simulink model "Hsp"  (Simulink 4.00)
settings: Solver=ode23t  StartTime=0  StopTime=70  FixedStep=0.01  RelTol=1e-3
PreLoadFcn:
  |  Control;HspInit;
values from neighbouring files (symbols this model uses):
  Cep = 1.67    [HspInit.m]    (also in hsp_data.mat)
  Cev = 50.0    (= 50)    [HspInit.m]    (also in hsp_data.mat)
  Cla = 19.23    [HspInit.m]    (also in hsp_data.mat)
  Cpa = 0.76    [HspInit.m]    (also in hsp_data.mat)
  Cpp = 5.80    (= 5.8)    [HspInit.m]    (also in hsp_data.mat)
  Cpv = 25.37    [HspInit.m]    (also in hsp_data.mat)
  Cra = 31.25    [HspInit.m]    (also in hsp_data.mat)
  Csa = 0.28    [HspInit.m]    (also in hsp_data.mat = 0.88)
  Csp = 2.05    [HspInit.m]    (also in hsp_data.mat)
  Csv = 61.11    [HspInit.m]    (also in hsp_data.mat)
  Dx = [  2     2     2     2    5      5        2   0.2 ]'    [Control.m]    (also in hsp_control.mat = [2 2 2 2 5 5 2 0.2])
  fcs0 = 25    [Control.m]    (also in hsp_control.mat)
  fes0 = 16.11    [Control.m]    (also in hsp_control.mat)
  fes1 = 2.10    (= 2.1)    [Control.m]    (also in hsp_control.mat)
  fesmin = 2.66    [Control.m]    (also in hsp_control.mat)
  fev0 = 3.2    [Control.m]    (also in hsp_control.mat)
  fev1 = 6.3    [Control.m]    (also in hsp_control.mat)
  fmax = 47.78    [Control.m]    (also in hsp_control.mat)
  fmin = 2.52    [Control.m]    (also in hsp_control.mat)
  Gx = [0.475 0.282  0.695 0.53 -265.4 -132.5  -0.13 0.09]'    [Control.m]    (also in hsp_control.mat = [0.475 0.282 0.695 0.53 -265.4 -132.5 -0.13 0.09])
  initx = [2.392 1.412  2.49  0.78 1435.4  1537    0.58   0]'    [Control.m]    (also in hsp_control.mat = [2.392 1.412 2.49 0.78 1400 1500 0.58 0])
  ka = 11.758    [Control.m]    (also in hsp_control.mat)
  KElv = 0.014    [HspInit.m]    (also in hsp_data.mat)
  KErv = 0.011    [HspInit.m]    (also in hsp_data.mat)
  kes = 0.0675    [Control.m]    (also in hsp_control.mat)
  kev = 7.06    [Control.m]    (also in hsp_control.mat)
  KRlv = 3.75e-4    (= 0.000375)    [HspInit.m]    (also in hsp_data.mat)
  KRrv = 1.4e-3    (= 0.0014)    [HspInit.m]    (also in hsp_data.mat)
  ksys = 0.075    [HspInit.m]    (also in hsp_data.mat)
  Lpa = 0.18e-3    (= 0.00018)    [HspInit.m]    (also in hsp_data.mat)
  Lsa = 0.22e-3    (= 0.00022)    [HspInit.m]    (also in hsp_data.mat)
  P0lv = 1.5    [HspInit.m]    (also in hsp_data.mat)
  P0rv = 1.5    [HspInit.m]    (also in hsp_data.mat)
  Pn = 92    [Control.m]    (also in hsp_control.mat)
  Rev = 0.016    [HspInit.m]    (also in hsp_data.mat)
  Rla = 25e-3    (= 0.025)    [HspInit.m]    (also in hsp_data.mat)
  Rpa = 0.023    [HspInit.m]    (also in hsp_data.mat)
  Rpp = 0.0894    [HspInit.m]    (also in hsp_data.mat)
  Rpv = 0.0056    [HspInit.m]    (also in hsp_data.mat)
  Rra = 2.5e-3    (= 0.0025)    [HspInit.m]    (also in hsp_data.mat)
  Rsa = 0.06    [HspInit.m]    (also in hsp_data.mat)
  Rsv = 0.038    [HspInit.m]    (also in hsp_data.mat)
  toup = 2.076    [Control.m]    (also in hsp_control.mat)
  toux = [  8     8     6     6    20     20       2   1.5 ]'    [Control.m]    (also in hsp_control.mat = [8 8 6 6 20 20 2 1.5])
  touz = 6.37    [Control.m]    (also in hsp_control.mat)
  Tsys0 = 0.5    [HspInit.m]    (also in hsp_data.mat)
  Vt = 5300    [HspInit.m]    (also in hsp_data.mat)
  Vuep = 336.6    [HspInit.m]    (also in hsp_data.mat)
  Vula = 25    [HspInit.m]    (also in hsp_data.mat)
  Vulv = 16.77    [HspInit.m]    (also in hsp_data.mat)
  Vupa = 0    [HspInit.m]    (also in hsp_data.mat)
  Vupp = 123    [HspInit.m]    (also in hsp_data.mat)
  Vupv = 120    [HspInit.m]    (also in hsp_data.mat)
  Vura = 25    [HspInit.m]    (also in hsp_data.mat)
  Vurv = 40.8    [HspInit.m]    (also in hsp_data.mat)
  Vusa = 0    [HspInit.m]    (also in hsp_data.mat)
  Vusp = 274.4    [HspInit.m]    (also in hsp_data.mat)
libraries: simulink3 x1
CloseFcn:
  | close(findobj(allchild(0),'flat','name','HSP Data Center'));close(findobj(allchild(0),'flat','name','HSP Control Center'))
settings Model: SaveOutput=off  InitialState=xFinal  SaveFinalState=on  LimitDataPoints=off  ExtModeTrigMode=oneshot  ExtModeArmWhenConnect=off  BlockReductionOpt=off

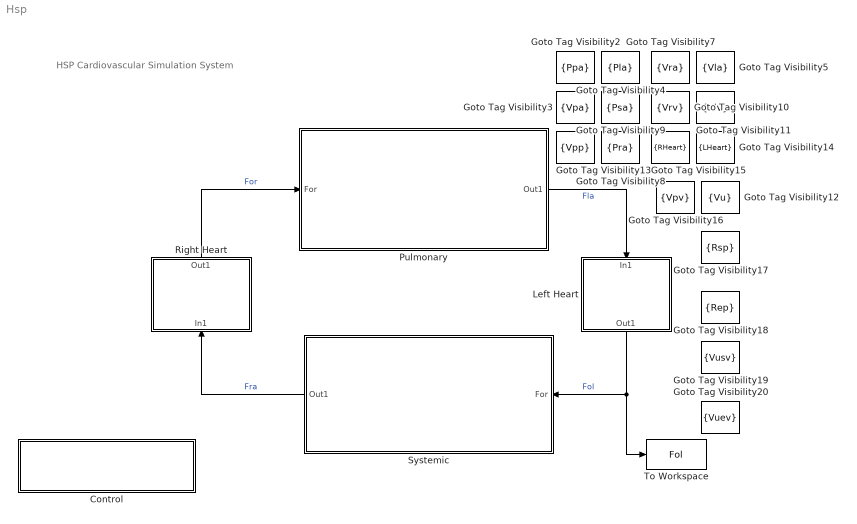
== system Hsp ==
  note: HSP
      | Cardiovascular Simulation System
  Control : Subsystem
      settings: RTWFcnNameOpts=Auto  RTWFileNameOpts=Auto
      mask Display: disp('ANALYSIS & CONTROL SYSTEM')
  Goto Tag Visibility10 : GotoTagVisibility  GotoTag=Vrv
  Goto Tag Visibility11 : GotoTagVisibility  GotoTag=Vlv
  Goto Tag Visibility12 : GotoTagVisibility  GotoTag=Vu
  Goto Tag Visibility13 : GotoTagVisibility  GotoTag=Vpp
  Goto Tag Visibility14 : GotoTagVisibility  GotoTag=LHeart
  Goto Tag Visibility15 : GotoTagVisibility  GotoTag=RHeart
  Goto Tag Visibility16 : GotoTagVisibility  GotoTag=Vpv
  Goto Tag Visibility17 : GotoTagVisibility  GotoTag=Rsp
  Goto Tag Visibility18 : GotoTagVisibility  GotoTag=Rep
  Goto Tag Visibility19 : GotoTagVisibility  GotoTag=Vusv
  Goto Tag Visibility2 : GotoTagVisibility  GotoTag=Ppa
  Goto Tag Visibility20 : GotoTagVisibility  GotoTag=Vuev
  Goto Tag Visibility3 : GotoTagVisibility  GotoTag=Vpa
  Goto Tag Visibility4 : GotoTagVisibility  GotoTag=Pla
  Goto Tag Visibility5 : GotoTagVisibility  GotoTag=Vla
  Goto Tag Visibility7 : GotoTagVisibility  GotoTag=Vra
  Goto Tag Visibility8 : GotoTagVisibility  GotoTag=Pra
  Goto Tag Visibility9 : GotoTagVisibility  GotoTag=Psa
  Left Heart : Subsystem  Orientation=down
      settings: RTWFcnNameOpts=Auto  RTWFileNameOpts=Auto
      mask Display: disp('LEFT HEART')
  Pulmonary : Subsystem
      settings: RTWFcnNameOpts=Auto  RTWFileNameOpts=Auto
      mask Display: disp('PULMONARY CIRCULATORY SYSTEM')
  Right Heart : Subsystem  Orientation=up
      settings: RTWFcnNameOpts=Auto  RTWFileNameOpts=Auto
      mask Display: disp('RIGHT HEART')
  Systemic : Subsystem  Orientation=left
      settings: RTWFcnNameOpts=Auto  RTWFileNameOpts=Auto
      mask Display: disp('SYSTEMIC CIRULATORY SYSTEM')
  To Workspace : ToWorkspace  VariableName=Fol  SampleTime=-1  SaveFormat=Array
  wires:
  Pulmonary/1(Out1) -> Left Heart/1(In1)  "Fla"
  Systemic/1(Out1) -> Right Heart/1(In1)  "Fra"
  Left Heart/1(Out1) -> Systemic/1(For), To Workspace/1  "Fol"
  Right Heart/1(Out1) -> Pulmonary/1(For)  "For"

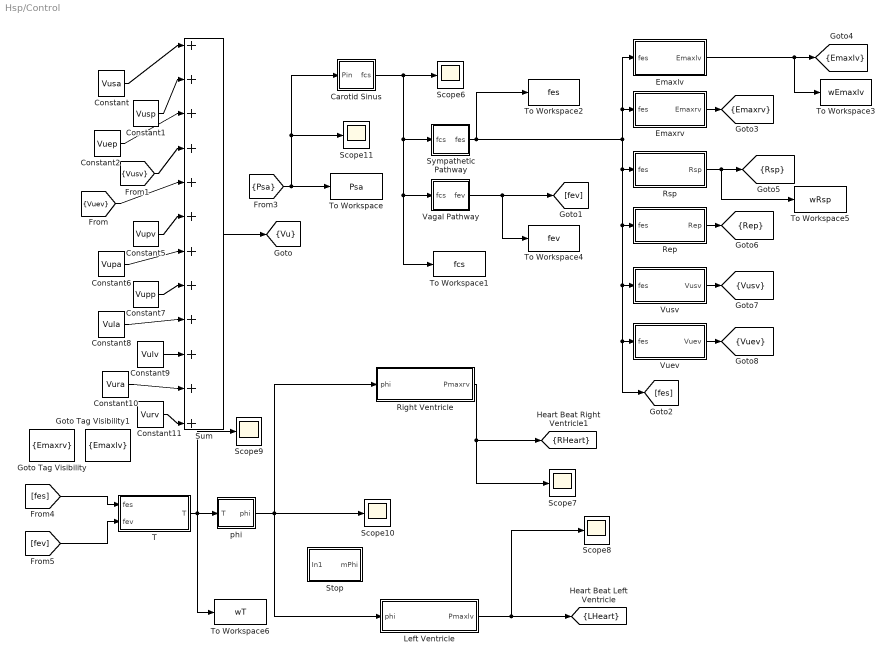
== system Hsp/Control ==
  Carotid Sinus : Subsystem
      settings: RTWFcnNameOpts=Auto  RTWFileNameOpts=Auto
  Constant : Constant  Value=Vusa
  Constant1 : Constant  Value=Vusp
  Constant10 : Constant  Value=Vura
  Constant11 : Constant  Value=Vurv
  Constant2 : Constant  Value=Vuep
  Constant5 : Constant  Value=Vupv
  Constant6 : Constant  Value=Vupa
  Constant7 : Constant  Value=Vupp
  Constant8 : Constant  Value=Vula
  Constant9 : Constant  Value=Vulv
  Emaxlv : Subsystem
      settings: RTWFcnNameOpts=Auto  RTWFileNameOpts=Auto
  Emaxrv : Subsystem
      settings: RTWFcnNameOpts=Auto  RTWFileNameOpts=Auto
  Goto Tag Visibility : GotoTagVisibility  GotoTag=Emaxrv
  Goto Tag Visibility1 : GotoTagVisibility  GotoTag=Emaxlv
  Left Ventricle : Subsystem
      settings: RTWFcnNameOpts=Auto  RTWFileNameOpts=Auto
  Rep : Subsystem
      settings: RTWFcnNameOpts=Auto  RTWFileNameOpts=Auto
  Right Ventricle : Subsystem
      settings: RTWFcnNameOpts=Auto  RTWFileNameOpts=Auto
  Rsp : Subsystem
      settings: RTWFcnNameOpts=Auto  RTWFileNameOpts=Auto
  Scope{6..11} (6 alike) : Scope
      Scope10 settings: TimeRange=auto  YMin=0  YMax=1  SaveToWorkspace=off  SaveName=ScopeData  LimitDataPoints=on  MaxDataPoints=5000
      Scope11 settings: TimeRange=auto  YMin=0  YMax=150  SaveToWorkspace=off  SaveName=ScopeData  LimitDataPoints=on  MaxDataPoints=5000
      Scope6 settings: TimeRange=auto  YMin=2.85  YMax=3.125  SaveToWorkspace=off  SaveName=ScopeData  LimitDataPoints=on  MaxDataPoints=5000
      Scope7 settings: TimeRange=auto  YMin=1.5  YMax=3.6  SaveToWorkspace=off  SaveName=ScopeData  LimitDataPoints=on  MaxDataPoints=5000
      Scope8 settings: TimeRange=auto  YMin=0  YMax=90  SaveToWorkspace=off  SaveName=ScopeData  LimitDataPoints=on  MaxDataPoints=5000
      Scope9 settings: TimeRange=auto  YMin=0.6  YMax=1.025  SaveToWorkspace=off  SaveName=ScopeData  LimitDataPoints=on  MaxDataPoints=5000
  Stop : Subsystem
      settings: RTWFcnNameOpts=Auto  RTWFileNameOpts=Auto
  Sum : Sum  Inputs=|++++++++++++  SaturateOnIntegerOverflow=on
  Sympathetic Pathway : Subsystem
      settings: RTWFcnNameOpts=Auto  RTWFileNameOpts=Auto
  T : Subsystem
      settings: RTWFcnNameOpts=Auto  RTWFileNameOpts=Auto
  To Workspace : ToWorkspace  VariableName=Psa  SampleTime=-1  SaveFormat=Array
  To Workspace1 : ToWorkspace  VariableName=fcs  SampleTime=-1  SaveFormat=Array
  To Workspace2 : ToWorkspace  VariableName=fes  SampleTime=-1  SaveFormat=Array
  To Workspace3 : ToWorkspace  VariableName=wEmaxlv  SampleTime=-1  SaveFormat=Array
  To Workspace4 : ToWorkspace  VariableName=fev  SampleTime=-1  SaveFormat=Array
  To Workspace5 : ToWorkspace  VariableName=wRsp  SampleTime=-1  SaveFormat=Array
  To Workspace6 : ToWorkspace  VariableName=wT  SampleTime=-1  SaveFormat=Array
  Vagal Pathway : Subsystem
      settings: RTWFcnNameOpts=Auto  RTWFileNameOpts=Auto
  Vuev : Subsystem
      settings: RTWFcnNameOpts=Auto  RTWFileNameOpts=Auto
  Vusv : Subsystem
      settings: RTWFcnNameOpts=Auto  RTWFileNameOpts=Auto
  phi : Subsystem
      settings: RTWFcnNameOpts=Auto  RTWFileNameOpts=Auto
  tag scope: Emaxlv=scoped, Emaxrv=scoped, LHeart=scoped, RHeart=scoped, Rep=scoped, Rsp=scoped, Vu=scoped, Vuev=scoped, Vusv=scoped
  wires:
  Sum/1 -> [Vu]
  Constant/1 -> Sum/1
  Constant2/1 -> Sum/3
  Constant1/1 -> Sum/2
  [Vusv] -> Sum/4
  [Vuev] -> Sum/5
  Constant5/1 -> Sum/6
  Constant6/1 -> Sum/7
  Constant7/1 -> Sum/8
  Constant8/1 -> Sum/9
  Constant9/1 -> Sum/10
  Constant10/1 -> Sum/11
  Constant11/1 -> Sum/12
  Carotid Sinus/1(fcs) -> Scope6/1, Sympathetic Pathway/1(fcs), Vagal Pathway/1(fcs), To Workspace1/1
  [fes] -> T/1(fes)
  [fev] -> T/2(fev)
  phi/1(phi) -> Scope10/1, Right Ventricle/1(phi), Left Ventricle/1(phi)
  Right Ventricle/1(Pmaxrv) -> [RHeart], Scope7/1
  Left Ventricle/1(Pmaxlv) -> [LHeart], Scope8/1
  Sympathetic Pathway/1(fes) -> Emaxlv/1(fes), Emaxrv/1(fes), Rsp/1(fes), Rep/1(fes), Vusv/1(fes), Vuev/1(fes), [fes], To Workspace2/1
  Emaxrv/1(Emaxrv) -> [Emaxrv]
  Rep/1(Rep) -> [Rep]
  Vusv/1(Vusv) -> [Vusv]
  Vuev/1(Vuev) -> [Vuev]
  Vagal Pathway/1(fev) -> [fev], To Workspace4/1
  Rsp/1(Rsp) -> [Rsp], To Workspace5/1
  [Psa] -> To Workspace/1, Scope11/1, Carotid Sinus/1(Pin)
  T/1(T) -> Scope9/1, To Workspace6/1, phi/1(T)
  Emaxlv/1(Emaxlv) -> [Emaxlv], To Workspace3/1

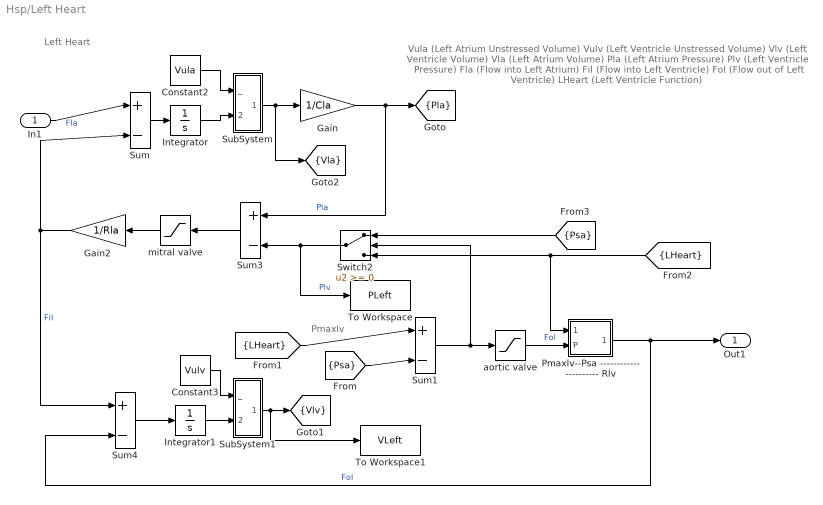
== system Hsp/Left Heart ==
  note: Left Heart
  note: Vula (Left Atrium Unstressed Volume)
      | Vulv (Left Ventricle Unstressed Volume)
      | Vlv (Left Ventricle Volume)
      | Vla (Left Atrium Volume)
      | Pla (Left Atrium Pressure)
      | Plv (Left Ventricle Pressure)
      | Fla (Flow into Left Atrium)
      | Fil (Flow into Left Ventricle)
      | Fol (Flow out of Left Ventricle)
      | LHeart (Left Ventricle Function)
  note: Pmaxlv
  In1 : Inport  Port=1
  Constant2 : Constant  Value=Vula
  Constant3 : Constant  Value=Vulv
  Gain : Gain  Gain=1/Cla  Multiplication=Element-wise(K.*u)  SaturateOnIntegerOverflow=on
  Gain2 : Gain  Orientation=left  Gain=1/Rla  Multiplication=Element-wise(K.*u)  SaturateOnIntegerOverflow=on
  Integrator : Integrator  ExternalReset=none  InitialConditionSource=internal  InitialCondition=0  LimitOutput=off  UpperSaturationLimit=inf  LowerSaturationLimit=-inf  ShowSaturationPort=off  ShowStatePort=off  AbsoluteTolerance=auto
  Integrator1 : Integrator  ExternalReset=none  InitialConditionSource=internal  InitialCondition=0  LimitOutput=off  UpperSaturationLimit=inf  LowerSaturationLimit=-inf  ShowSaturationPort=off  ShowStatePort=off  AbsoluteTolerance=auto
  Pmaxlv--Psa ---------------------- Rlv : Subsystem
      settings: RTWFcnNameOpts=Auto  RTWFileNameOpts=Auto
  SubSystem : Subsystem
      settings: RTWFcnNameOpts=Auto  RTWFileNameOpts=Auto
  SubSystem1 : Subsystem
      settings: RTWFcnNameOpts=Auto  RTWFileNameOpts=Auto
  Sum : Sum  Inputs=|+-  SaturateOnIntegerOverflow=on
  Sum1 : Sum  Inputs=|+-  SaturateOnIntegerOverflow=on
  Sum3 : Sum  Orientation=left  Inputs=+-  SaturateOnIntegerOverflow=on
  Sum4 : Sum  Inputs=+-  SaturateOnIntegerOverflow=on
  Switch2 : Switch  Orientation=left  Threshold=0
  To Workspace : ToWorkspace  VariableName=PLeft  SampleTime=-1  SaveFormat=Array
  To Workspace1 : ToWorkspace  VariableName=VLeft  SampleTime=-1  SaveFormat=Array
  aortic valve : Saturate  UpperLimit=inf  LowerLimit=0  LinearizeAsGain=on
  mitral valve : Saturate  Orientation=left  UpperLimit=inf  LowerLimit=0  LinearizeAsGain=on
  Out1 : Outport  Port=1
  tag scope: Pla=scoped, Vla=scoped, Vlv=scoped
  wires:
  In1/1 -> Sum/1  "Fla"
  Sum/1 -> Integrator/1
  [Psa] -> Sum1/2
  Gain/1 -> [Pla], Sum3/1  "Pla"
  Sum4/1 -> Integrator1/1
  Gain2/1 -> Sum/2, Sum4/1  "Fil"
  Pmaxlv--Psa ---------------------- Rlv/1(Flow) -> Out1/1, Sum4/2  "Fol"
  Constant2/1 -> SubSystem/1(_)
  Constant3/1 -> SubSystem1/1(_)
  SubSystem/1(Out) -> Gain/1, [Vla]
  [LHeart] -> Sum1/1
  Sum1/1 -> aortic valve/1, Switch2/2
  [Psa] -> Switch2/1
  mitral valve/1 -> Gain2/1
  [LHeart] -> Switch2/3, Pmaxlv--Psa ---------------------- Rlv/1(Pmax)
  aortic valve/1 -> Pmaxlv--Psa ---------------------- Rlv/2(P)  "Fol"
  Switch2/1 -> Sum3/2, To Workspace/1  "Plv"
  SubSystem1/1(Out) -> [Vlv], To Workspace1/1
  Integrator1/1 -> SubSystem1/2(+)
  Sum3/1 -> mitral valve/1
  Integrator/1 -> SubSystem/2(+)

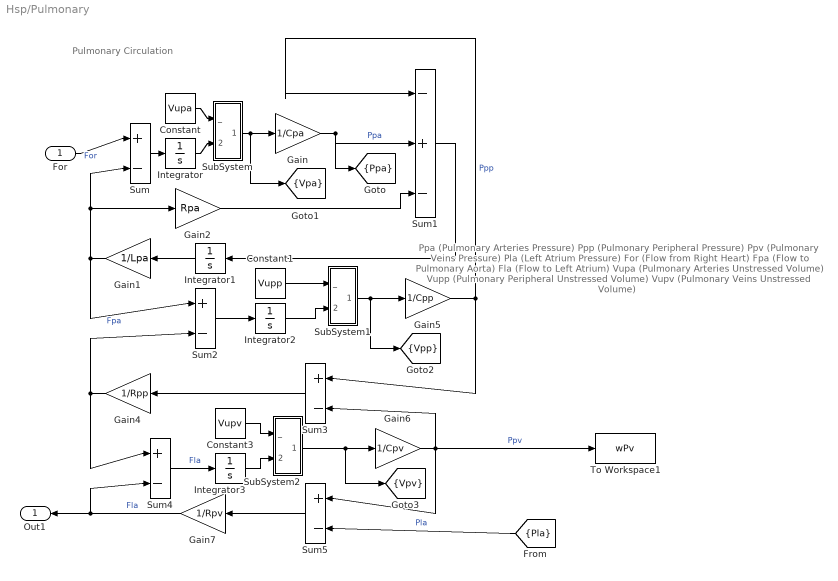
== system Hsp/Pulmonary ==
  note: Ppa (Pulmonary Arteries Pressure)
      | Ppp (Pulmonary Peripheral Pressure)
      | Ppv (Pulmonary Veins Pressure)
      | Pla (Left Atrium Pressure)
      | For (Flow from Right Heart)
      | Fpa (Flow to Pulmonary Aorta)
      | Fla (Flow to Left Atrium)
      | Vupa (Pulmonary Arteries Unstressed Volume)
      | Vupp (Pulmonary Peripheral Unstressed Volume)
      | Vupv (Pulmonary Veins Unstressed Volume)
  note: Pulmonary Circulation
  For : Inport  Port=1
  Constant : Constant  Value=Vupa
  Constant1 : Constant  Value=Vupp
  Constant3 : Constant  Value=Vupv
  Gain : Gain  Gain=1/Cpa  Multiplication=Element-wise(K.*u)  SaturateOnIntegerOverflow=on
  Gain1 : Gain  Orientation=left  Gain=1/Lpa  Multiplication=Element-wise(K.*u)  SaturateOnIntegerOverflow=on
  Gain2 : Gain  Gain=Rpa  Multiplication=Element-wise(K.*u)  SaturateOnIntegerOverflow=on
  Gain4 : Gain  Orientation=left  Gain=1/Rpp  Multiplication=Element-wise(K.*u)  SaturateOnIntegerOverflow=on
  Gain5 : Gain  Gain=1/Cpp  Multiplication=Element-wise(K.*u)  SaturateOnIntegerOverflow=on
  Gain6 : Gain  Gain=1/Cpv  Multiplication=Element-wise(K.*u)  SaturateOnIntegerOverflow=on
  Gain7 : Gain  Orientation=left  Gain=1/Rpv  Multiplication=Element-wise(K.*u)  SaturateOnIntegerOverflow=on
  Integrator : Integrator  ExternalReset=none  InitialConditionSource=internal  InitialCondition=100  LimitOutput=off  UpperSaturationLimit=inf  LowerSaturationLimit=-inf  ShowSaturationPort=off  ShowStatePort=off  AbsoluteTolerance=auto
  Integrator1 : Integrator  Orientation=left  ExternalReset=none  InitialConditionSource=internal  InitialCondition=0  LimitOutput=off  UpperSaturationLimit=inf  LowerSaturationLimit=-inf  ShowSaturationPort=off  ShowStatePort=off  AbsoluteTolerance=auto
  Integrator2 : Integrator  ExternalReset=none  InitialConditionSource=internal  InitialCondition=100  LimitOutput=off  UpperSaturationLimit=inf  LowerSaturationLimit=-inf  ShowSaturationPort=off  ShowStatePort=off  AbsoluteTolerance=auto
  Integrator3 : Integrator  ExternalReset=none  InitialConditionSource=internal  InitialCondition=0  LimitOutput=off  UpperSaturationLimit=inf  LowerSaturationLimit=-inf  ShowSaturationPort=off  ShowStatePort=off  AbsoluteTolerance=auto
  SubSystem : Subsystem
      settings: RTWFcnNameOpts=Auto  RTWFileNameOpts=Auto
  SubSystem1 : Subsystem
      settings: RTWFcnNameOpts=Auto  RTWFileNameOpts=Auto
  SubSystem2 : Subsystem
      settings: RTWFcnNameOpts=Auto  RTWFileNameOpts=Auto
  Sum : Sum  Inputs=|+-  SaturateOnIntegerOverflow=on
  Sum1 : Sum  Inputs=|-+-  SaturateOnIntegerOverflow=on
  Sum2 : Sum  Inputs=|+-  SaturateOnIntegerOverflow=on
  Sum3 : Sum  Orientation=left  Inputs=|+-  SaturateOnIntegerOverflow=on
  Sum4 : Sum  Inputs=|+-  SaturateOnIntegerOverflow=on
  Sum5 : Sum  Orientation=left  Inputs=|+-  SaturateOnIntegerOverflow=on
  To Workspace1 : ToWorkspace  VariableName=wPv  SampleTime=-1  SaveFormat=Array
  Out1 : Outport  Orientation=left  Port=1
  tag scope: Ppa=scoped, Vpa=scoped, Vpp=scoped, Vpv=scoped
  wires:
  For/1 -> Sum/1  "For"
  Sum/1 -> Integrator/1
  Integrator1/1 -> Gain1/1
  Sum1/1 -> Integrator1/1
  Gain2/1 -> Sum1/3
  Gain1/1 -> Sum/2, Gain2/1, Sum2/1  "Fpa"
  Sum2/1 -> Integrator2/1
  Gain5/1 -> Sum1/1, Sum3/1  "Ppp"
  Sum3/1 -> Gain4/1
  Gain4/1 -> Sum2/2, Sum4/1
  Sum5/1 -> Gain7/1
  Gain6/1 -> Sum3/2, Sum5/1, To Workspace1/1  "Ppv"
  [Pla] -> Sum5/2  "Pla"
  Sum4/1 -> Integrator3/1  "Fla"
  Gain/1 -> Sum1/2, [Ppa]  "Ppa"
  SubSystem/1(Out) -> Gain/1, [Vpa]
  SubSystem1/1(Out) -> Gain5/1, [Vpp]
  SubSystem2/1(Out) -> Gain6/1, [Vpv]
  Integrator/1 -> SubSystem/2(+)
  Constant/1 -> SubSystem/1(_)
  Constant1/1 -> SubSystem1/1(_)
  Integrator2/1 -> SubSystem1/2(+)
  Integrator3/1 -> SubSystem2/2(+)
  Gain7/1 -> Sum4/2, Out1/1  "Fla"
  Constant3/1 -> SubSystem2/1(_)

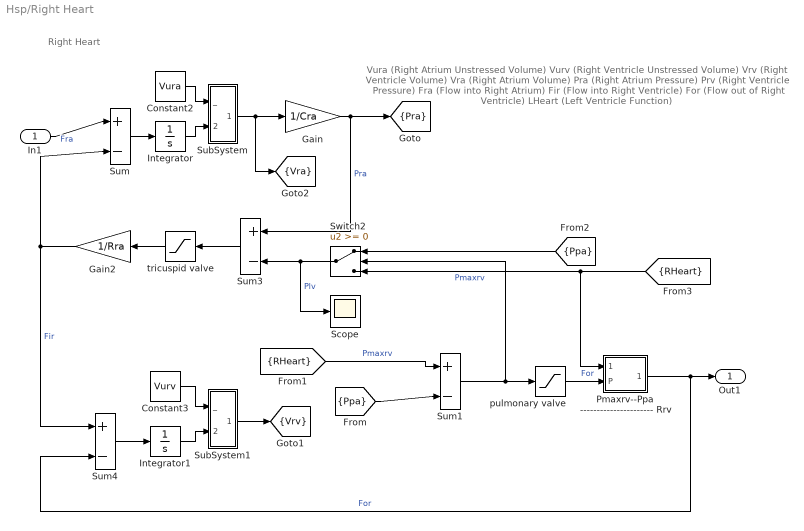
== system Hsp/Right Heart ==
  note: Right Heart
  note: Vura (Right Atrium Unstressed Volume)
      | Vurv (Right Ventricle Unstressed Volume)
      | Vrv (Right Ventricle Volume)
      | Vra (Right Atrium Volume)
      | Pra (Right Atrium Pressure)
      | Prv (Right Ventricle Pressure)
      | Fra (Flow into Right Atrium)
      | Fir (Flow into Right Ventricle)
      | For (Flow out of Right Ventricle)
      | LHeart (Left Ventricle Function)
  In1 : Inport  Port=1
  Constant2 : Constant  Value=Vura
  Constant3 : Constant  Value=Vurv
  Gain : Gain  Gain=1/Cra  Multiplication=Element-wise(K.*u)  SaturateOnIntegerOverflow=on
  Gain2 : Gain  Orientation=left  Gain=1/Rra  Multiplication=Element-wise(K.*u)  SaturateOnIntegerOverflow=on
  Integrator : Integrator  ExternalReset=none  InitialConditionSource=internal  InitialCondition=0  LimitOutput=off  UpperSaturationLimit=inf  LowerSaturationLimit=-inf  ShowSaturationPort=off  ShowStatePort=off  AbsoluteTolerance=auto
  Integrator1 : Integrator  ExternalReset=none  InitialConditionSource=internal  InitialCondition=0  LimitOutput=off  UpperSaturationLimit=inf  LowerSaturationLimit=-inf  ShowSaturationPort=off  ShowStatePort=off  AbsoluteTolerance=auto
  Pmaxrv--Ppa ---------------------- Rrv : Subsystem
      settings: RTWFcnNameOpts=Auto  RTWFileNameOpts=Auto
  Scope : Scope
      settings: TimeRange=auto  YMin=125  YMax=160  SaveToWorkspace=off  SaveName=ScopeData  LimitDataPoints=on  MaxDataPoints=5000
  SubSystem : Subsystem
      settings: RTWFcnNameOpts=Auto  RTWFileNameOpts=Auto
  SubSystem1 : Subsystem
      settings: RTWFcnNameOpts=Auto  RTWFileNameOpts=Auto
  Sum : Sum  Inputs=|+-  SaturateOnIntegerOverflow=on
  Sum1 : Sum  Inputs=|+-  SaturateOnIntegerOverflow=on
  Sum3 : Sum  Orientation=left  Inputs=+-  SaturateOnIntegerOverflow=on
  Sum4 : Sum  Inputs=+-  SaturateOnIntegerOverflow=on
  Switch2 : Switch  Orientation=left  Threshold=0
  pulmonary valve : Saturate  UpperLimit=inf  LowerLimit=0  LinearizeAsGain=on
  tricuspid valve : Saturate  Orientation=left  UpperLimit=inf  LowerLimit=0  LinearizeAsGain=on
  Out1 : Outport  Port=1
  tag scope: Pra=scoped, Vra=scoped, Vrv=scoped
  wires:
  In1/1 -> Sum/1  "Fra"
  Sum/1 -> Integrator/1
  [Ppa] -> Sum1/2
  Gain/1 -> [Pra], Sum3/1  "Pra"
  Gain2/1 -> Sum/2, Sum4/1  "Fir"
  Integrator/1 -> SubSystem/2(+)
  Constant2/1 -> SubSystem/1(_)
  SubSystem1/1(Out) -> [Vrv]
  SubSystem/1(Out) -> Gain/1, [Vra]
  Constant3/1 -> SubSystem1/1(_)
  Integrator1/1 -> SubSystem1/2(+)
  [RHeart] -> Sum1/1  "Pmaxrv"
  Sum1/1 -> pulmonary valve/1, Switch2/2
  [Ppa] -> Switch2/1
  tricuspid valve/1 -> Gain2/1
  pulmonary valve/1 -> Pmaxrv--Ppa ---------------------- Rrv/2(P)  "For"
  Pmaxrv--Ppa ---------------------- Rrv/1(Flow) -> Out1/1, Sum4/2  "For"
  [RHeart] -> Switch2/3, Pmaxrv--Ppa ---------------------- Rrv/1(Pmax)  "Pmaxrv"
  Sum4/1 -> Integrator1/1
  Sum3/1 -> tricuspid valve/1
  Switch2/1 -> Sum3/2, Scope/1  "Plv"

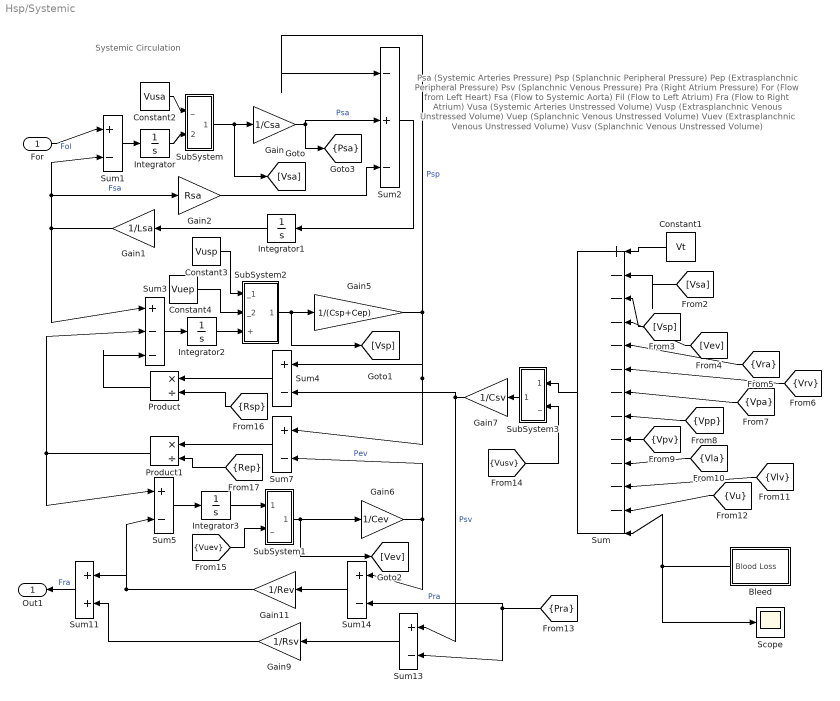
== system Hsp/Systemic ==
  note: Psa (Systemic Arteries Pressure)
      | Psp (Splanchnic Peripheral Pressure)
      | Pep (Extrasplanchnic Peripheral Pressure)
      | Psv (Splanchnic Venous Pressure)
      | Pra (Right Atrium Pressure)
      | For (Flow from Left Heart)
      | Fsa (Flow to Systemic Aorta)
      | Fil (Flow to Left Atrium)
      | Fra (Flow to Right Atrium)
      | Vusa (Systemic Arteries Unstressed Volume)
      | Vusp (Extrasplanchnic Venous Unstressed Volume)
      | Vuep (Splanchnic Venous Unstressed Volume)
      | Vuev (Extrasplanchnic Venous Unstressed Volume)
      | Vusv (Splanchnic Venous Unstressed Volume)
  note: Systemic Circulation
  For : Inport  Port=1
  Bleed : Subsystem  Orientation=left  mask{ulimit=0, rate=0, tstart=0}
      mask prompts: ulimit "Bleed Up Limit (ml)"; rate "Bleed Rate (ml/s)"; tstart "Bleed Start Time (s)"
      settings: RTWFcnNameOpts=Auto  RTWFileNameOpts=Auto
  Constant1 : Constant  Orientation=left  Value=Vt
  Constant2 : Constant  Value=Vusa
  Constant3 : Constant  Value=Vusp
  Constant4 : Constant  Value=Vuep
  Gain : Gain  Gain=1/Csa  Multiplication=Element-wise(K.*u)  SaturateOnIntegerOverflow=on
  Gain1 : Gain  Orientation=left  Gain=1/Lsa  Multiplication=Element-wise(K.*u)  SaturateOnIntegerOverflow=on
  Gain11 : Gain  Orientation=left  Gain=1/Rev  Multiplication=Element-wise(K.*u)  SaturateOnIntegerOverflow=on
  Gain2 : Gain  Gain=Rsa  Multiplication=Element-wise(K.*u)  SaturateOnIntegerOverflow=on
  Gain5 : Gain  Gain=1/(Csp+Cep)  Multiplication=Element-wise(K.*u)  SaturateOnIntegerOverflow=on
  Gain6 : Gain  Gain=1/Cev  Multiplication=Element-wise(K.*u)  SaturateOnIntegerOverflow=on
  Gain7 : Gain  Orientation=left  Gain=1/Csv  Multiplication=Element-wise(K.*u)  SaturateOnIntegerOverflow=on
  Gain9 : Gain  Orientation=left  Gain=1/Rsv  Multiplication=Element-wise(K.*u)  SaturateOnIntegerOverflow=on
  Integrator : Integrator  ExternalReset=none  InitialConditionSource=internal  InitialCondition=0  LimitOutput=off  UpperSaturationLimit=inf  LowerSaturationLimit=-inf  ShowSaturationPort=off  ShowStatePort=off  AbsoluteTolerance=auto
  Integrator1 : Integrator  Orientation=left  ExternalReset=none  InitialConditionSource=internal  InitialCondition=0  LimitOutput=off  UpperSaturationLimit=inf  LowerSaturationLimit=-inf  ShowSaturationPort=off  ShowStatePort=off  AbsoluteTolerance=auto
  Integrator2 : Integrator  ExternalReset=none  InitialConditionSource=internal  InitialCondition=0  LimitOutput=off  UpperSaturationLimit=inf  LowerSaturationLimit=-inf  ShowSaturationPort=off  ShowStatePort=off  AbsoluteTolerance=auto
  Integrator3 : Integrator  ExternalReset=none  InitialConditionSource=internal  InitialCondition=0  LimitOutput=off  UpperSaturationLimit=inf  LowerSaturationLimit=-inf  ShowSaturationPort=off  ShowStatePort=off  AbsoluteTolerance=auto
  Product : Product  Orientation=left  Inputs=*/  Multiplication=Element-wise(.*)  SaturateOnIntegerOverflow=on
  Product1 : Product  Orientation=left  Inputs=*/  Multiplication=Element-wise(.*)  SaturateOnIntegerOverflow=on
  Scope : Scope
      settings: TimeRange=auto  YMin=0  YMax=200  SaveToWorkspace=off  SaveName=ScopeData  LimitDataPoints=on  MaxDataPoints=5000
  SubSystem : Subsystem
      settings: RTWFcnNameOpts=Auto  RTWFileNameOpts=Auto
  SubSystem1 : Subsystem
      settings: RTWFcnNameOpts=Auto  RTWFileNameOpts=Auto
  SubSystem2 : Subsystem
      settings: RTWFcnNameOpts=Auto  RTWFileNameOpts=Auto
  SubSystem3 : Subsystem  Orientation=left
      settings: RTWFcnNameOpts=Auto  RTWFileNameOpts=Auto
  Sum : Sum  Orientation=left  Inputs=|+------------  SaturateOnIntegerOverflow=on
  Sum1 : Sum  Inputs=|+-  SaturateOnIntegerOverflow=on
  Sum11 : Sum  Orientation=left  Inputs=|++  SaturateOnIntegerOverflow=on
  Sum{4,7,13..14} (4 alike) : Sum  Orientation=left  Inputs=|+-  SaturateOnIntegerOverflow=on
  Sum2 : Sum  Inputs=|-+-  SaturateOnIntegerOverflow=on
  Sum3 : Sum  Inputs=|+--  SaturateOnIntegerOverflow=on
  Sum5 : Sum  Inputs=|+-  SaturateOnIntegerOverflow=on
  Out1 : Outport  Orientation=left  Port=1
  tag scope: Psa=scoped
  wires:
  For/1 -> Sum1/1  "Fol"
  Sum1/1 -> Integrator/1
  Integrator1/1 -> Gain1/1
  Sum2/1 -> Integrator1/1
  Gain2/1 -> Sum2/3
  Gain1/1 -> Sum1/2, Gain2/1, Sum3/1  "Fsa"
  Sum3/1 -> Integrator2/1
  Gain5/1 -> Sum2/1, Sum4/1, Sum7/1  "Psp"
  Product/1 -> Sum3/3
  Product1/1 -> Sum3/2, Sum5/1
  Integrator3/1 -> SubSystem1/1(+)
  SubSystem1/1(Out) -> Gain6/1, [Vev]
  Constant1/1 -> Sum/1
  [Vsa] -> Sum/2
  [Vsp] -> Sum/3
  [Vev] -> Sum/4
  [Vra] -> Sum/5
  [Vrv] -> Sum/6
  [Vpa] -> Sum/7
  [Vpp] -> Sum/8
  [Vpv] -> Sum/9
  [Vla] -> Sum/10
  [Vlv] -> Sum/11
  [Vu] -> Sum/12
  Integrator/1 -> SubSystem/2(+)
  SubSystem/1(Out) -> Gain/1, [Vsa]
  Integrator2/1 -> SubSystem2/3(+)
  SubSystem2/1(Out) -> Gain5/1, [Vsp]
  SubSystem3/1(Out) -> Gain7/1
  Sum13/1 -> Gain9/1
  Sum11/1 -> Out1/1  "Fra"
  Gain7/1 -> Sum4/2, Sum13/1  "Psv"
  Gain9/1 -> Sum11/2
  Gain6/1 -> Sum7/2, Sum14/1  "Pev"
  Sum14/1 -> Gain11/1
  [Pra] -> Sum13/2, Sum14/2  "Pra"
  Sum5/1 -> Integrator3/1
  Gain11/1 -> Sum11/1, Sum5/2
  Gain/1 -> Sum2/2, [Psa]  "Psa"
  Constant2/1 -> SubSystem/1(_)
  [Vuev] -> SubSystem1/2(_)
  Constant3/1 -> SubSystem2/1(_1)
  Constant4/1 -> SubSystem2/2(_2)
  Sum/1 -> SubSystem3/1(+)
  [Vusv] -> SubSystem3/2(_)
  Sum4/1 -> Product/1
  [Rsp] -> Product/2
  [Rep] -> Product1/2
  Sum7/1 -> Product1/1
  Bleed/1(Blood Loss) -> Sum/13, Scope/1

== system Hsp/Control/Carotid Sinus ==
  Pin : Inport  Port=1
  Fcn : Fcn  Expr=(fmin+fmax*exp((u-Pn)/ka))/(1+exp((u-Pn)/ka))
  Transfer Fcn : TransferFcn  Numerator=[touz 1]  Denominator=[toup 1]  Realization=auto  AbsoluteTolerance=auto
  fcs : Outport  Port=1
  wires:
  Pin/1 -> Transfer Fcn/1
  Transfer Fcn/1 -> Fcn/1
  Fcn/1 -> fcs/1

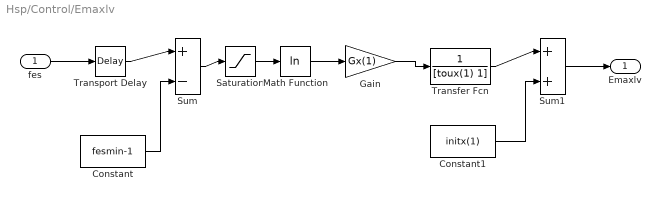
== system Hsp/Control/Emaxlv ==
  fes : Inport  Port=1
  Constant : Constant  Value=fesmin-1
  Constant1 : Constant  Value=initx(1)
  Gain : Gain  Gain=Gx(1)  Multiplication=Element-wise(K.*u)  SaturateOnIntegerOverflow=on
  Math Function : Math  Operator=log  OutputSignalType=auto
  Saturation : Saturate  UpperLimit=inf  LowerLimit=1  LinearizeAsGain=on
  Sum : Sum  Inputs=|+-  SaturateOnIntegerOverflow=on
  Sum1 : Sum  Inputs=|++  SaturateOnIntegerOverflow=on
  Transfer Fcn : TransferFcn  Numerator=[1]  Denominator=[toux(1) 1]  Realization=auto  AbsoluteTolerance=auto
  Transport Delay : TransportDelay  DelayTime=Dx(1)  InitialInput=0  BufferSize=1024  PadeOrder=0
  Emaxlv : Outport  Port=1
  wires:
  fes/1 -> Transport Delay/1
  Transport Delay/1 -> Sum/1
  Constant/1 -> Sum/2
  Sum/1 -> Saturation/1
  Saturation/1 -> Math Function/1
  Math Function/1 -> Gain/1
  Gain/1 -> Transfer Fcn/1
  Transfer Fcn/1 -> Sum1/1
  Sum1/1 -> Emaxlv/1
  Constant1/1 -> Sum1/2

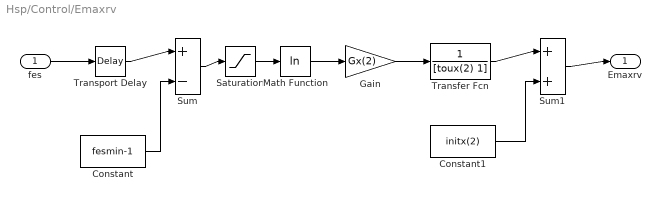
== system Hsp/Control/Emaxrv ==
  fes : Inport  Port=1
  Constant : Constant  Value=fesmin-1
  Constant1 : Constant  Value=initx(2)
  Gain : Gain  Gain=Gx(2)  Multiplication=Element-wise(K.*u)  SaturateOnIntegerOverflow=on
  Math Function : Math  Operator=log  OutputSignalType=auto
  Saturation : Saturate  UpperLimit=inf  LowerLimit=1  LinearizeAsGain=on
  Sum : Sum  Inputs=|+-  SaturateOnIntegerOverflow=on
  Sum1 : Sum  Inputs=|++  SaturateOnIntegerOverflow=on
  Transfer Fcn : TransferFcn  Numerator=[1]  Denominator=[toux(2) 1]  Realization=auto  AbsoluteTolerance=auto
  Transport Delay : TransportDelay  DelayTime=Dx(2)  InitialInput=0  BufferSize=1024  PadeOrder=0
  Emaxrv : Outport  Port=1
  wires:
  Constant1/1 -> Sum1/2
  Sum1/1 -> Emaxrv/1
  Transfer Fcn/1 -> Sum1/1
  Gain/1 -> Transfer Fcn/1
  Math Function/1 -> Gain/1
  Saturation/1 -> Math Function/1
  Sum/1 -> Saturation/1
  Constant/1 -> Sum/2
  Transport Delay/1 -> Sum/1
  fes/1 -> Transport Delay/1

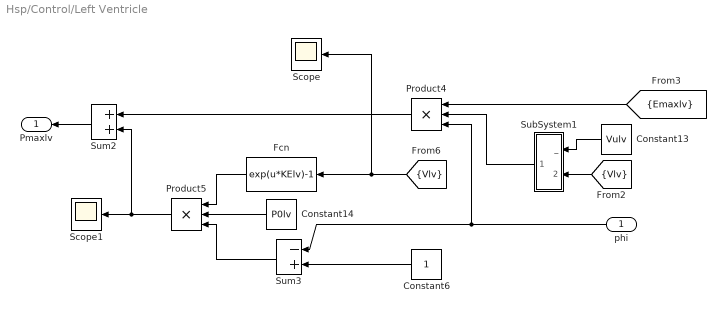
== system Hsp/Control/Left Ventricle ==
  phi : Inport  Orientation=left  Port=1
  Constant13 : Constant  Orientation=left  Value=Vulv
  Constant14 : Constant  Orientation=left  Value=P0lv
  Constant6 : Constant  Orientation=left  Value=1
  Fcn : Fcn  Orientation=left  Expr=exp(u*KElv)-1
  Product4 : Product  Orientation=left  Inputs=3  Multiplication=Element-wise(.*)  SaturateOnIntegerOverflow=on
  Product5 : Product  Orientation=left  Inputs=3  Multiplication=Element-wise(.*)  SaturateOnIntegerOverflow=on
  Scope : Scope
      settings: TimeRange=auto  YMin=0  YMax=250  SaveToWorkspace=off  SaveName=ScopeData  LimitDataPoints=on  MaxDataPoints=5000
  Scope1 : Scope
      settings: TimeRange=auto  YMin=0  YMax=35  SaveToWorkspace=off  LimitDataPoints=on  MaxDataPoints=5000
  SubSystem1 : Subsystem  Orientation=left
      settings: RTWFcnNameOpts=Auto  RTWFileNameOpts=Auto
  Sum2 : Sum  Orientation=left  Inputs=++  SaturateOnIntegerOverflow=on
  Sum3 : Sum  Orientation=left  Inputs=-+  SaturateOnIntegerOverflow=on
  Pmaxlv : Outport  Orientation=left  Port=1
  wires:
  Sum2/1 -> Pmaxlv/1
  Product4/1 -> Sum2/1
  Product5/1 -> Sum2/2, Scope1/1
  Fcn/1 -> Product5/1
  Constant14/1 -> Product5/2
  Sum3/1 -> Product5/3
  Constant6/1 -> Sum3/2
  Constant13/1 -> SubSystem1/1(_)
  [Vlv] -> SubSystem1/2(+)
  SubSystem1/1(Out) -> Product4/2
  phi/1 -> Sum3/1, Product4/3
  [Emaxlv] -> Product4/1
  [Vlv] -> Fcn/1, Scope/1

== system Hsp/Control/Rep ==
  fes : Inport  Port=1
  Constant : Constant  Value=fesmin-1
  Constant1 : Constant  Value=initx(4)
  Gain : Gain  Gain=Gx(4)  Multiplication=Element-wise(K.*u)  SaturateOnIntegerOverflow=on
  Math Function : Math  Operator=log  OutputSignalType=auto
  Saturation : Saturate  UpperLimit=inf  LowerLimit=1  LinearizeAsGain=on
  Sum : Sum  Inputs=|+-  SaturateOnIntegerOverflow=on
  Sum1 : Sum  Inputs=|++  SaturateOnIntegerOverflow=on
  Transfer Fcn : TransferFcn  Numerator=[1]  Denominator=[toux(4) 1]  Realization=auto  AbsoluteTolerance=auto
  Transport Delay : TransportDelay  DelayTime=Dx(4)  InitialInput=0  BufferSize=1024  PadeOrder=0
  Rep : Outport  Port=1
  wires:
  Constant1/1 -> Sum1/2
  Sum1/1 -> Rep/1
  Transfer Fcn/1 -> Sum1/1
  Gain/1 -> Transfer Fcn/1
  Math Function/1 -> Gain/1
  Saturation/1 -> Math Function/1
  Sum/1 -> Saturation/1
  Constant/1 -> Sum/2
  Transport Delay/1 -> Sum/1
  fes/1 -> Transport Delay/1

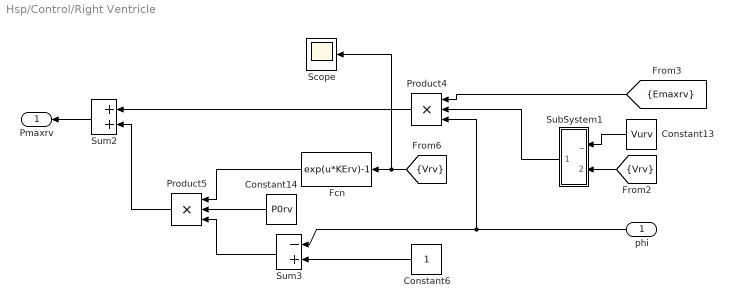
== system Hsp/Control/Right Ventricle ==
  phi : Inport  Orientation=left  Port=1
  Constant13 : Constant  Orientation=left  Value=Vurv
  Constant14 : Constant  Orientation=left  Value=P0rv
  Constant6 : Constant  Orientation=left  Value=1
  Fcn : Fcn  Orientation=left  Expr=exp(u*KErv)-1
  Product4 : Product  Orientation=left  Inputs=3  Multiplication=Element-wise(.*)  SaturateOnIntegerOverflow=on
  Product5 : Product  Orientation=left  Inputs=3  Multiplication=Element-wise(.*)  SaturateOnIntegerOverflow=on
  Scope : Scope
      settings: TimeRange=auto  YMin=45  YMax=85  SaveToWorkspace=off  SaveName=ScopeData  LimitDataPoints=on  MaxDataPoints=5000
  SubSystem1 : Subsystem  Orientation=left
      settings: RTWFcnNameOpts=Auto  RTWFileNameOpts=Auto
  Sum2 : Sum  Orientation=left  Inputs=++  SaturateOnIntegerOverflow=on
  Sum3 : Sum  Orientation=left  Inputs=-+  SaturateOnIntegerOverflow=on
  Pmaxrv : Outport  Orientation=left  Port=1
  wires:
  Constant6/1 -> Sum3/2
  Sum3/1 -> Product5/3
  Constant14/1 -> Product5/2
  Fcn/1 -> Product5/1
  Product5/1 -> Sum2/2
  Product4/1 -> Sum2/1
  Sum2/1 -> Pmaxrv/1
  [Emaxrv] -> Product4/1
  [Vrv] -> SubSystem1/2(+)
  Constant13/1 -> SubSystem1/1(_)
  SubSystem1/1(Out) -> Product4/2
  phi/1 -> Sum3/1, Product4/3
  [Vrv] -> Fcn/1, Scope/1

== system Hsp/Control/Rsp ==
  fes : Inport  Port=1
  Constant : Constant  Value=fesmin-1
  Constant1 : Constant  Value=initx(3)
  Gain : Gain  Gain=Gx(3)  Multiplication=Element-wise(K.*u)  SaturateOnIntegerOverflow=on
  Math Function : Math  Operator=log  OutputSignalType=auto
  Saturation : Saturate  UpperLimit=inf  LowerLimit=1  LinearizeAsGain=on
  Sum : Sum  Inputs=|+-  SaturateOnIntegerOverflow=on
  Sum1 : Sum  Inputs=|++  SaturateOnIntegerOverflow=on
  Transfer Fcn : TransferFcn  Numerator=[1]  Denominator=[toux(3) 1]  Realization=auto  AbsoluteTolerance=auto
  Transport Delay : TransportDelay  DelayTime=Dx(3)  InitialInput=0  BufferSize=1024  PadeOrder=0
  Rsp : Outport  Port=1
  wires:
  fes/1 -> Transport Delay/1
  Transport Delay/1 -> Sum/1
  Constant/1 -> Sum/2
  Sum/1 -> Saturation/1
  Saturation/1 -> Math Function/1
  Math Function/1 -> Gain/1
  Gain/1 -> Transfer Fcn/1
  Transfer Fcn/1 -> Sum1/1
  Sum1/1 -> Rsp/1
  Constant1/1 -> Sum1/2

== system Hsp/Control/Stop ==
  In1 : Inport  Port=1
  Clock : Clock
      settings: DisplayTime=off  Decimation=10
  Constant : Constant  Value=0
  Switch : Switch  Threshold=50
  mPhi : Outport  Port=1
  wires:
  In1/1 -> Switch/3
  Constant/1 -> Switch/1
  Switch/1 -> mPhi/1
  Clock/1 -> Switch/2

== system Hsp/Control/Sympathetic Pathway ==
  fcs : Inport  Port=1
  Constant : Constant  Value=fes1
  Gain : Gain  Gain=-kes  Multiplication=Element-wise(K.*u)  SaturateOnIntegerOverflow=on
  Gain1 : Gain  Gain=fes0-fes1  Multiplication=Element-wise(K.*u)  SaturateOnIntegerOverflow=on
  Math Function : Math  Operator=exp  OutputSignalType=auto
  Sum : Sum  Inputs=|++  SaturateOnIntegerOverflow=on
  fes : Outport  Port=1
  wires:
  Gain1/1 -> Sum/1
  Constant/1 -> Sum/2
  Sum/1 -> fes/1
  fcs/1 -> Gain/1
  Gain/1 -> Math Function/1
  Math Function/1 -> Gain1/1

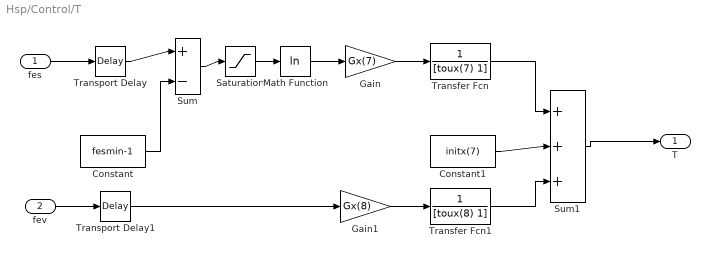
== system Hsp/Control/T ==
  fes : Inport  Port=1
  fev : Inport  Port=2
  Constant : Constant  Value=fesmin-1
  Constant1 : Constant  Value=initx(7)
  Gain : Gain  Gain=Gx(7)  Multiplication=Element-wise(K.*u)  SaturateOnIntegerOverflow=on
  Gain1 : Gain  Gain=Gx(8)  Multiplication=Element-wise(K.*u)  SaturateOnIntegerOverflow=on
  Math Function : Math  Operator=log  OutputSignalType=auto
  Saturation : Saturate  UpperLimit=inf  LowerLimit=1  LinearizeAsGain=on
  Sum : Sum  Inputs=|+-  SaturateOnIntegerOverflow=on
  Sum1 : Sum  Inputs=|+++  SaturateOnIntegerOverflow=on
  Transfer Fcn : TransferFcn  Numerator=[1]  Denominator=[toux(7) 1]  Realization=auto  AbsoluteTolerance=auto
  Transfer Fcn1 : TransferFcn  Numerator=[1]  Denominator=[toux(8) 1]  Realization=auto  AbsoluteTolerance=auto
  Transport Delay : TransportDelay  DelayTime=Dx(7)  InitialInput=0  BufferSize=1024  PadeOrder=0
  Transport Delay1 : TransportDelay  DelayTime=Dx(8)  InitialInput=0  BufferSize=1024  PadeOrder=0
  T : Outport  Port=1
  wires:
  fes/1 -> Transport Delay/1
  Transport Delay/1 -> Sum/1
  Constant/1 -> Sum/2
  Sum/1 -> Saturation/1
  Saturation/1 -> Math Function/1
  Math Function/1 -> Gain/1
  Gain/1 -> Transfer Fcn/1
  Transfer Fcn/1 -> Sum1/1
  Sum1/1 -> T/1
  Constant1/1 -> Sum1/2
  fev/1 -> Transport Delay1/1
  Transport Delay1/1 -> Gain1/1
  Gain1/1 -> Transfer Fcn1/1
  Transfer Fcn1/1 -> Sum1/3

== system Hsp/Control/Vagal Pathway ==
  fcs : Inport  Port=1
  Fcn : Fcn  Expr=(fev0+fev1*exp((u-fcs0)/kev))/(1+exp((u-fcs0)/kev))
  fev : Outport  Port=1
  wires:
  Fcn/1 -> fev/1
  fcs/1 -> Fcn/1

== system Hsp/Control/Vuev ==
  fes : Inport  Port=1
  Constant : Constant  Value=fesmin-1
  Constant1 : Constant  Value=initx(6)
  Gain : Gain  Gain=Gx(6)  Multiplication=Element-wise(K.*u)  SaturateOnIntegerOverflow=on
  Math Function : Math  Operator=log  OutputSignalType=auto
  Saturation : Saturate  UpperLimit=inf  LowerLimit=1  LinearizeAsGain=on
  Sum : Sum  Inputs=|+-  SaturateOnIntegerOverflow=on
  Sum1 : Sum  Inputs=|++  SaturateOnIntegerOverflow=on
  Transfer Fcn : TransferFcn  Numerator=[1]  Denominator=[toux(6) 1]  Realization=auto  AbsoluteTolerance=auto
  Transport Delay : TransportDelay  DelayTime=Dx(6)  InitialInput=0  BufferSize=1024  PadeOrder=0
  Vuev : Outport  Port=1
  wires:
  Constant1/1 -> Sum1/2
  Sum1/1 -> Vuev/1
  Transfer Fcn/1 -> Sum1/1
  Gain/1 -> Transfer Fcn/1
  Math Function/1 -> Gain/1
  Saturation/1 -> Math Function/1
  Sum/1 -> Saturation/1
  Constant/1 -> Sum/2
  Transport Delay/1 -> Sum/1
  fes/1 -> Transport Delay/1

== system Hsp/Control/Vusv ==
  fes : Inport  Port=1
  Constant : Constant  Value=fesmin-1
  Constant1 : Constant  Value=initx(5)
  Gain : Gain  Gain=Gx(5)  Multiplication=Element-wise(K.*u)  SaturateOnIntegerOverflow=on
  Math Function : Math  Operator=log  OutputSignalType=auto
  Saturation : Saturate  UpperLimit=inf  LowerLimit=1  LinearizeAsGain=on
  Sum : Sum  Inputs=|+-  SaturateOnIntegerOverflow=on
  Sum1 : Sum  Inputs=|++  SaturateOnIntegerOverflow=on
  Transfer Fcn : TransferFcn  Numerator=[1]  Denominator=[toux(5) 1]  Realization=auto  AbsoluteTolerance=auto
  Transport Delay : TransportDelay  DelayTime=Dx(5)  InitialInput=0  BufferSize=1024  PadeOrder=0
  Vusv : Outport  Port=1
  wires:
  fes/1 -> Transport Delay/1
  Transport Delay/1 -> Sum/1
  Constant/1 -> Sum/2
  Sum/1 -> Saturation/1
  Saturation/1 -> Math Function/1
  Math Function/1 -> Gain/1
  Gain/1 -> Transfer Fcn/1
  Transfer Fcn/1 -> Sum1/1
  Sum1/1 -> Vusv/1
  Constant1/1 -> Sum1/2

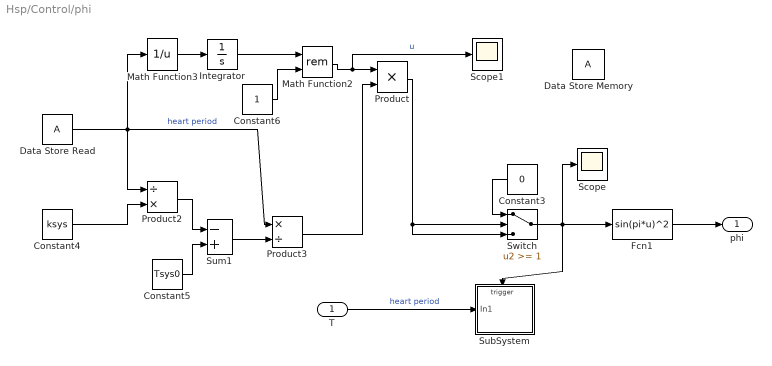
== system Hsp/Control/phi ==
  T : Inport  Port=1
  Constant3 : Constant  Orientation=left  Value=0
  Constant4 : Constant  Value=ksys
  Constant5 : Constant  Value=Tsys0
  Constant6 : Constant  Value=1
  Data Store Memory : DataStoreMemory  DataStoreName=A  InitialValue=initx(7)
  Data Store Read : DataStoreRead  DataStoreName=A  SampleTime=0
  Fcn1 : Fcn  Expr=sin(pi*u)^2
  Integrator : Integrator  ExternalReset=none  InitialConditionSource=internal  InitialCondition=0  LimitOutput=off  UpperSaturationLimit=inf  LowerSaturationLimit=-inf  ShowSaturationPort=off  ShowStatePort=off  AbsoluteTolerance=auto
  Math Function2 : Math  Operator=rem  OutputSignalType=auto
  Math Function3 : Math  Operator=reciprocal  OutputSignalType=auto
  Product : Product  Inputs=2  Multiplication=Element-wise(.*)  SaturateOnIntegerOverflow=on
  Product2 : Product  Inputs=/*  Multiplication=Element-wise(.*)  SaturateOnIntegerOverflow=on
  Product3 : Product  Inputs=*/  Multiplication=Element-wise(.*)  SaturateOnIntegerOverflow=on
  Scope : Scope
      settings: TimeRange=auto  YMin=0  YMax=1  SaveToWorkspace=off  SaveName=ScopeData  LimitDataPoints=on  MaxDataPoints=5000
  Scope1 : Scope
      settings: TimeRange=auto  YMin=5.55112e-017  YMax=1  SaveToWorkspace=off  SaveName=ScopeData  LimitDataPoints=on  MaxDataPoints=5000
  SubSystem : Subsystem  TreatAsAtomicUnit=on
      settings: RTWFcnNameOpts=Auto  RTWFileNameOpts=Auto
  Sum1 : Sum  Inputs=-+  SaturateOnIntegerOverflow=on
  Switch : Switch  Threshold=1
  phi : Outport  Port=1
  wires:
  Product3/1 -> Product/2
  Sum1/1 -> Product3/2
  Constant5/1 -> Sum1/2
  Product2/1 -> Sum1/1
  Constant4/1 -> Product2/2
  Constant3/1 -> Switch/1
  Product/1 -> Switch/2, Switch/3
  Fcn1/1 -> phi/1
  T/1 -> SubSystem/1(In1)  "heart period"
  Switch/1 -> Fcn1/1, SubSystem/Trigger, Scope/1
  Data Store Read/1 -> Product3/1, Product2/1, Math Function3/1  "heart period"
  Constant6/1 -> Math Function2/2
  Math Function2/1 -> Product/1, Scope1/1  "u"
  Math Function3/1 -> Integrator/1
  Integrator/1 -> Math Function2/1

== system Hsp/Left Heart/Pmaxlv--Psa ---------------------- Rlv ==
  Pmax : Inport  Port=1
  P : Inport  Port=2
  Gain : Gain  Gain=KRlv  Multiplication=Element-wise(K.*u)  SaturateOnIntegerOverflow=on
  Product : Product  Inputs=/*  Multiplication=Element-wise(.*)  SaturateOnIntegerOverflow=on
  Saturation : Saturate  UpperLimit=inf  LowerLimit=0.01  LinearizeAsGain=on
  Flow : Outport  Port=1
  wires:
  Pmax/1 -> Gain/1
  Gain/1 -> Saturation/1
  P/1 -> Product/2
  Saturation/1 -> Product/1
  Product/1 -> Flow/1

== system Hsp/Left Heart/SubSystem ==
  _ : Inport  Port=1
  + : Inport  Port=2
  Saturation : Saturate  UpperLimit=10000  LowerLimit=0  LinearizeAsGain=on
  Sum : Sum  Inputs=|-+  SaturateOnIntegerOverflow=on
  Out : Outport  Port=1
  wires:
  _/1 -> Sum/1
  +/1 -> Sum/2
  Sum/1 -> Saturation/1
  Saturation/1 -> Out/1

== system Hsp/Left Heart/SubSystem1 ==
  _ : Inport  Port=1
  + : Inport  Port=2
  Saturation : Saturate  UpperLimit=10000  LowerLimit=0  LinearizeAsGain=on
  Sum : Sum  Inputs=|-+  SaturateOnIntegerOverflow=on
  Out : Outport  Port=1
  wires:
  Saturation/1 -> Out/1
  Sum/1 -> Saturation/1
  +/1 -> Sum/2
  _/1 -> Sum/1

== system Hsp/Pulmonary/SubSystem ==
  _ : Inport  Port=1
  + : Inport  Port=2
  Saturation : Saturate  UpperLimit=10000  LowerLimit=0  LinearizeAsGain=on
  Sum : Sum  Inputs=|-+  SaturateOnIntegerOverflow=on
  Out : Outport  Port=1
  wires:
  _/1 -> Sum/1
  +/1 -> Sum/2
  Sum/1 -> Saturation/1
  Saturation/1 -> Out/1

== system Hsp/Pulmonary/SubSystem1 ==
  _ : Inport  Port=1
  + : Inport  Port=2
  Saturation : Saturate  UpperLimit=10000  LowerLimit=0  LinearizeAsGain=on
  Sum : Sum  Inputs=|-+  SaturateOnIntegerOverflow=on
  Out : Outport  Port=1
  wires:
  _/1 -> Sum/1
  +/1 -> Sum/2
  Sum/1 -> Saturation/1
  Saturation/1 -> Out/1

== system Hsp/Pulmonary/SubSystem2 ==
  _ : Inport  Port=1
  + : Inport  Port=2
  Saturation : Saturate  UpperLimit=10000  LowerLimit=0  LinearizeAsGain=on
  Sum : Sum  Inputs=|-+  SaturateOnIntegerOverflow=on
  Out : Outport  Port=1
  wires:
  Saturation/1 -> Out/1
  Sum/1 -> Saturation/1
  +/1 -> Sum/2
  _/1 -> Sum/1

== system Hsp/Right Heart/Pmaxrv--Ppa ---------------------- Rrv ==
  Pmax : Inport  Port=1
  P : Inport  Port=2
  Gain : Gain  Gain=KRrv  Multiplication=Element-wise(K.*u)  SaturateOnIntegerOverflow=on
  Product : Product  Inputs=/*  Multiplication=Element-wise(.*)  SaturateOnIntegerOverflow=on
  Saturation : Saturate  UpperLimit=inf  LowerLimit=0.01  LinearizeAsGain=on
  Flow : Outport  Port=1
  wires:
  Pmax/1 -> Gain/1
  Gain/1 -> Saturation/1
  P/1 -> Product/2
  Saturation/1 -> Product/1
  Product/1 -> Flow/1

== system Hsp/Right Heart/SubSystem ==
  _ : Inport  Port=1
  + : Inport  Port=2
  Saturation : Saturate  UpperLimit=10000  LowerLimit=0  LinearizeAsGain=on
  Sum : Sum  Inputs=|-+  SaturateOnIntegerOverflow=on
  Out : Outport  Port=1
  wires:
  _/1 -> Sum/1
  +/1 -> Sum/2
  Sum/1 -> Saturation/1
  Saturation/1 -> Out/1

== system Hsp/Right Heart/SubSystem1 ==
  _ : Inport  Port=1
  + : Inport  Port=2
  Saturation : Saturate  UpperLimit=10000  LowerLimit=0  LinearizeAsGain=on
  Sum : Sum  Inputs=|-+  SaturateOnIntegerOverflow=on
  Out : Outport  Port=1
  wires:
  Saturation/1 -> Out/1
  Sum/1 -> Saturation/1
  +/1 -> Sum/2
  _/1 -> Sum/1

== system Hsp/Systemic/Bleed ==
  Clock : Clock
      settings: DisplayTime=off  Decimation=10
  Constant : Constant  Value=0
  Ramp : simulink3/Sources/Ramp  slope=rate  start=tstart  X0=0
  Saturation : Saturate  UpperLimit=ulimit  LowerLimit=0  LinearizeAsGain=on
  Switch : Switch  Threshold=tstart
  Blood Loss : Outport  Port=1
  wires:
  Clock/1 -> Switch/2
  Constant/1 -> Switch/3
  Ramp/1 -> Switch/1
  Switch/1 -> Saturation/1
  Saturation/1 -> Blood Loss/1

== system Hsp/Systemic/SubSystem ==
  _ : Inport  Port=1
  + : Inport  Port=2
  Saturation : Saturate  UpperLimit=10000  LowerLimit=0  LinearizeAsGain=on
  Sum : Sum  Inputs=|-+  SaturateOnIntegerOverflow=on
  Out : Outport  Port=1
  wires:
  _/1 -> Sum/1
  +/1 -> Sum/2
  Sum/1 -> Saturation/1
  Saturation/1 -> Out/1

== system Hsp/Systemic/SubSystem1 ==
  + : Inport  Port=1
  _ : Inport  Port=2
  Saturation : Saturate  UpperLimit=10000  LowerLimit=0  LinearizeAsGain=on
  Sum : Sum  Inputs=|+-  SaturateOnIntegerOverflow=on
  Out : Outport  Port=1
  wires:
  Saturation/1 -> Out/1
  Sum/1 -> Saturation/1
  _/1 -> Sum/2
  +/1 -> Sum/1

== system Hsp/Systemic/SubSystem2 ==
  _1 : Inport  Port=1
  _2 : Inport  Port=2
  + : Inport  Port=3
  Saturation : Saturate  UpperLimit=10000  LowerLimit=0  LinearizeAsGain=on
  Sum : Sum  Inputs=|--+  SaturateOnIntegerOverflow=on
  Out : Outport  Port=1
  wires:
  Saturation/1 -> Out/1
  Sum/1 -> Saturation/1
  _1/1 -> Sum/1
  +/1 -> Sum/3
  _2/1 -> Sum/2

== system Hsp/Systemic/SubSystem3 ==
  + : Inport  Port=1
  _ : Inport  Port=2
  Saturation : Saturate  UpperLimit=10000  LowerLimit=0  LinearizeAsGain=on
  Sum : Sum  Inputs=|+-  SaturateOnIntegerOverflow=on
  Out : Outport  Port=1
  wires:
  +/1 -> Sum/1
  _/1 -> Sum/2
  Sum/1 -> Saturation/1
  Saturation/1 -> Out/1

== system Hsp/Control/Left Ventricle/SubSystem1 ==
  _ : Inport  Port=1
  + : Inport  Port=2
  Saturation : Saturate  UpperLimit=10000  LowerLimit=0  LinearizeAsGain=on
  Sum : Sum  Inputs=|-+  SaturateOnIntegerOverflow=on
  Out : Outport  Port=1
  wires:
  _/1 -> Sum/1
  +/1 -> Sum/2
  Sum/1 -> Saturation/1
  Saturation/1 -> Out/1

== system Hsp/Control/Right Ventricle/SubSystem1 ==
  _ : Inport  Port=1
  + : Inport  Port=2
  Saturation : Saturate  UpperLimit=10000  LowerLimit=0  LinearizeAsGain=on
  Sum : Sum  Inputs=|-+  SaturateOnIntegerOverflow=on
  Out : Outport  Port=1
  wires:
  Saturation/1 -> Out/1
  Sum/1 -> Saturation/1
  +/1 -> Sum/2
  _/1 -> Sum/1

== system Hsp/Control/phi/SubSystem ==
  In1 : Inport  Port=1
  Trigger : TriggerPort  TriggerType=rising  OutputDataType=auto
  Data Store Write : DataStoreWrite  DataStoreName=A  SampleTime=-1
  Scope : Scope
      settings: TimeRange=auto  YMin=-5  YMax=5  SaveToWorkspace=off  SaveName=ScopeData  LimitDataPoints=on  MaxDataPoints=5000
  wires:
  In1/1 -> Data Store Write/1, Scope/1
